simulink model "victim_detector"  (Simulink 8.7)
settings: Solver=FixedStepAuto  StartTime=0.0  StopTime=10.0  RelTol=1e-3
settings Model: Creator=eispin  LastModifiedBy=eispin
settings DataIOCC: LimitDataPoints=off  SaveFormat=Dataset
settings DebuggingCC: UnderspecifiedInitializationDetection=Simplified  MergeDetectMultiDrivingBlocksExec=error
settings HardwareCC: ProdBitPerPointer=64  ProdLargestAtomicFloat=Float  ProdIntDivRoundTo=Zero  ProdEndianess=LittleEndian  ProdWordSize=64  ProdHWDeviceType=Intel->x86-64 (Windows64)
settings ModelReferenceCC: PropagateSignalLabelsOutOfModel=on
settings ConfigComp: CovModelRefEnable=off

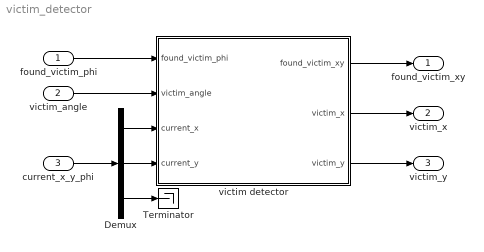
== system victim_detector ==
  found_victim_phi : Inport
  victim_angle : Inport  Port=2  OutDataTypeStr=double
  current_x_y_phi : Inport  Port=3
  Demux : Demux  Outputs=3
  Terminator : Terminator
  victim detector : Stateflow chart  TreatAsAtomicUnit=on
  found_victim_xy : Outport
  victim_x : Outport  Port=2
  victim_y : Outport  Port=3
  wires:
  found_victim_phi/1 -> victim detector/1(found_victim_phi)
  victim_angle/1 -> victim detector/2(victim_angle)
  victim detector/1(found_victim_xy) -> found_victim_xy/1
  victim detector/2(victim_x) -> victim_x/1
  victim detector/3(victim_y) -> victim_y/1
  Demux/1 -> victim detector/3(current_x)
  Demux/2 -> victim detector/4(current_y)
  Demux/3 -> Terminator/1
  current_x_y_phi/1 -> Demux/1

== stateflow chart victim detector ==
  state WaitForNewInformation
  state EnoughInformationAboutVictim
    entry:
    information(1,2) = information(1,1);
    information(2,2) = information(2,1);
    information(3,2) = information(3,1);
    information(1,1) = current_x;
    information(2,1) = current_y;
    information(3,1) = victim_angle;
    [computed_victim_x, computed_victim_y] = compute_position(information);
    if computed_victim_x >= 1 && computed_victim_x <= 200 && computed_victim_y >= 1 && computed_victim_y <= 200
    victim_x = computed_victim_x;
    victim_y = computed_victim_y;
    found_victim_xy = 1;
    end;
  state NoInformationAboutVictim
    entry:
    found_victim_xy = 0;
    %row 1: x, row 2: y, row 3: phi
    information = zeros(3, 2);
  state SomeInformationAboutVictim
    entry:
    information(1,1) = current_x;
    information(2,1) = current_y;
    information(3,1) = victim_angle;
  (default) -> NoInformationAboutVictim
  NoInformationAboutVictim -> SomeInformationAboutVictim : [found_victim_phi == 1]
  SomeInformationAboutVictim -> WaitForNewInformation : [found_victim_phi == 0]
  WaitForNewInformation -> EnoughInformationAboutVictim : [found_victim_phi == 1]
  EnoughInformationAboutVictim -> WaitForNewInformation : [found_victim_phi == 0]
  data: info function_input double; x function_output double; y function_output double; found_victim_xy output double; victim_x output double; victim_y output double; found_victim_phi input double; victim_angle input double; current_x input double; current_y input double; information local double; computed_victim_x local double; computed_victim_y local double
  function [x, y] = compute_position(info):
    | function [x, y] = compute_position(info)
    |     v1 = [cos(info(3,1)) sin(info(3,1))];
    |     v1_orth = cross2d(v1);
    |     v2 = [cos(info(3,2)) sin(info(3,2))];
    |     v2_orth = cross2d(v2);
    |     o1 = [info(1,1); info(2,1)];
    |     o2 = [info(1,2); info(2,2)];
    | 
    |     M = [v1_orth; v2_orth];
    |     b = [v1_orth*o1; v2_orth*o2];
    |     xy = mldivide(M, b); % Solve equation system: M * xy = b
    |     x = xy(1);
    |     y = xy(2);
    | 
    |     % Sanity check
    |     if v1_orth * ([x; y] - o1) >= 0.1 ...
    |             || v2_orth * ([x; y] - o2) >= 0.1
    |         x = -1;
    |         y = -1;
    |     end
    | end
    | 
    | function v = cross2d(v)
    |     % The cross product in 2d is unary
    |     v = [-v(2) v(1)];
    | end
